simulink model "FlexibleJoint_NNO"  (R2021a)
settings: Solver=VariableStepAuto  StartTime=0.0  StopTime=100  RelTol=1e-3
values from neighbouring files (symbols this model uses):
  A = [[-20 1;0 -20] zeros(2);zeros(2) [-20 1;0 -20]]    [parameters.m]
  Ac = A - G*C    [parameters.m]
  C = eye(4)    [parameters.m]
  eta1 = 1000    [parameters.m]
  eta2 = 1000    [parameters.m]
  G = place(A',C',poles_desired)'    [parameters.m]
  rho1 = 1.5    [parameters.m]
  rho2 = 1.5    [parameters.m]
  size_hiddenlayerneurons = 5    [parameters.m]
  size_systeminput = 1    [parameters.m]
  V0 = 0.1*(2*rand(size_hiddenlayerneurons,size_states + size_systeminput))+100    [parameters.m]
  W0 = 0.1*(2*rand(size_states,size_hiddenlayerneurons))+10    [parameters.m]
settings Model: Creator=kiankhaneghahi  LastModifiedBy=kiankhaneghahi

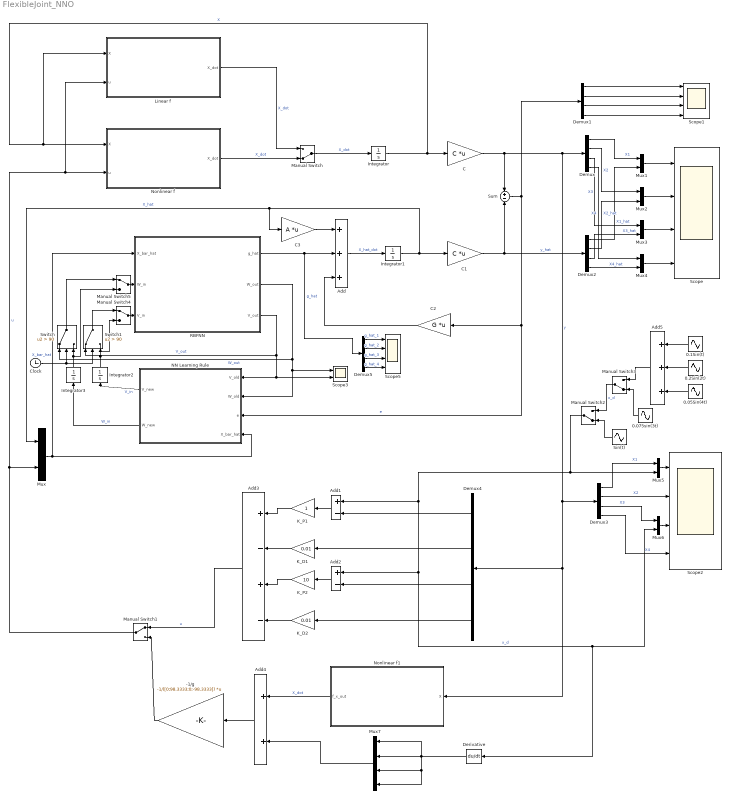
== system FlexibleJoint_NNO ==
  -1/g : Gain  Gain=-1/([0;98.3333;0;-98.3333])  Multiplication=Matrix(K*u)
  0.05Sin(4t) : Sin  Amplitude=0.05  Frequency=4  SampleTime=0
  0.075sin(3t) : Sin  Amplitude=0.075  Frequency=3  SampleTime=0
  0.1Sin(t) : Sin  Amplitude=0.1  SampleTime=0
  0.2Sin(2t) : Sin  Amplitude=0.2  Frequency=2  SampleTime=0
  Add : Sum  Inputs=+++
  Add1 : Sum  Inputs=+-
  Add2 : Sum  Inputs=+-
  Add3 : Sum  Inputs=+-+-
  Add4 : Sum
  Add5 : Sum  Inputs=+++
  C : Gain  Gain=C  Multiplication=Matrix(K*u)
  C1 : Gain  Gain=C  Multiplication=Matrix(K*u)
  C2 : Gain  Gain=G  Multiplication=Matrix(K*u)
  C3 : Gain  Gain=A  Multiplication=Matrix(K*u)
  Clock : Clock
  Demux{,1..5} (6 alike) : Demux
  Derivative : Derivative
  Integrator : Integrator  InitialCondition=[0;0;0;0]
  Integrator1 : Integrator  InitialCondition=[0;0;0;0]
  Integrator2 : Integrator  InitialCondition=V0
  Integrator3 : Integrator  InitialCondition=W0
  K_D1 : Gain  Gain=0.01
  K_D2 : Gain  Gain=0.01
  K_P1 : Gain
  K_P2 : Gain  Gain=10
  Linear f : MATLAB Function  TreatAsAtomicUnit=on
  Manual Switch : ManualSwitch  CurrentSetting=0
  Manual Switch1 : ManualSwitch
  Manual Switch2 : ManualSwitch  CurrentSetting=0
  Manual Switch3 : ManualSwitch  CurrentSetting=0
  Manual Switch4 : ManualSwitch
  Manual Switch5 : ManualSwitch
  Mux{,1..6} (7 alike) : Mux  Inputs=2
  Mux7 : Mux
  NN Learning Rule : MATLAB Function  TreatAsAtomicUnit=on
  Nonlinear f : MATLAB Function  TreatAsAtomicUnit=on
  Nonlinear f1 : MATLAB Function  TreatAsAtomicUnit=on
  RBFNN : MATLAB Function  TreatAsAtomicUnit=on
  Scope{,1..2,5} (4 alike) : Scope  NumInputPorts=4
  Scope3 : Scope  NumInputPorts=2
  Sin(t) : Sin  SampleTime=0
  Sum : Sum  Inputs=+-
  Switch : Switch  Criteria=u2 > Threshold  Threshold=90
  Switch1 : Switch  Criteria=u2 > Threshold  Threshold=90
  wires:
  Integrator/1 -> Linear f/1(X), Nonlinear f/1(X), C/1  "X"
  C3/1 -> Add/1
  NN Learning Rule/1(V_new) -> Integrator2/1  "V_in"
  NN Learning Rule/2(W_new) -> Integrator3/1  "W_in"
  Mux/1 -> NN Learning Rule/4(X_bar_hat), RBFNN/1(X_bar_hat)  "X_bar_hat"
  C1/1 -> Demux2/1, Sum/2  "y_hat"
  Integrator1/1 -> C3/1, Mux/1, C1/1  "X_hat"
  C2/1 -> Add/3
  RBFNN/2(W_out) -> Switch/1, NN Learning Rule/2(W_old), Scope3/1  "W_out"
  Add/1 -> Integrator1/1  "X_hat_dot"
  RBFNN/1(g_hat) -> Demux5/1, Add/2  "g_hat"
  Sum/1 -> Demux1/1, C2/1, NN Learning Rule/3(e)  "e"
  RBFNN/3(V_out) -> NN Learning Rule/1(V_old), Scope3/2, Switch1/1  "V_out"
  C/1 -> Demux4/1, Nonlinear f1/1(X), Demux3/1, Demux/1, Sum/1  "y"
  Manual Switch1/1 -> Linear f/2(u), Nonlinear f/2(u), Mux/2  "u"
  Manual Switch/1 -> Integrator/1  "X_dot"
  Nonlinear f/1(X_dot) -> Manual Switch/2  "X_dot"
  Linear f/1(X_dot) -> Manual Switch/1  "X_dot"
  Demux1/1 -> Scope1/1
  Demux1/2 -> Scope1/2
  Demux1/3 -> Scope1/3
  Demux1/4 -> Scope1/4
  Mux1/1 -> Scope/1
  Mux2/1 -> Scope/2
  Mux3/1 -> Scope/3
  Mux4/1 -> Scope/4
  Demux/1 -> Mux1/1  "X1"
  Demux2/1 -> Mux1/2  "X1_hat"
  Demux/2 -> Mux2/1  "X2"
  Demux2/2 -> Mux2/2  "X2_hat"
  Demux/3 -> Mux3/1  "X3"
  Demux2/3 -> Mux3/2  "X3_hat"
  Demux2/4 -> Mux4/2  "X4_hat"
  Demux/4 -> Mux4/1  "X4"
  Demux3/1 -> Mux5/1  "X1"
  Demux3/2 -> Scope2/2  "X2"
  Demux3/3 -> Mux6/1  "X3"
  Demux3/4 -> Scope2/4  "X4"
  Add1/1 -> K_P1/1
  Demux4/1 -> Add1/2
  Demux4/3 -> Add2/2
  Add2/1 -> K_P2/1
  Demux4/2 -> K_D1/1
  Demux4/4 -> K_D2/1
  K_D1/1 -> Add3/2
  K_D2/1 -> Add3/4
  K_P1/1 -> Add3/1
  K_P2/1 -> Add3/3
  Manual Switch4/1 -> RBFNN/3(V_in)
  Manual Switch5/1 -> RBFNN/2(W_in)
  Mux5/1 -> Scope2/1
  Mux6/1 -> Scope2/3
  Demux5/1 -> Scope5/1  "g_hat_1"
  Demux5/2 -> Scope5/2  "g_hat_2"
  Demux5/3 -> Scope5/3  "g_hat_3"
  Demux5/4 -> Scope5/4  "g_hat_4"
  Add3/1 -> Manual Switch1/1  "u"
  Nonlinear f1/1(f_x_out) -> Add4/1  "X_dot"
  Add4/1 -> -1/g/1
  -1/g/1 -> Manual Switch1/2
  Derivative/1 -> Mux7/3, Mux7/4, Mux7/2, Mux7/1
  Mux7/1 -> Add4/2
  Manual Switch2/1 -> Mux5/2, Derivative/1, Mux6/2, Add2/1, Add1/1  "x_d"
  Sin(t)/1 -> Manual Switch2/2
  Manual Switch3/1 -> Manual Switch2/1  "x_d"
  0.075sin(3t)/1 -> Manual Switch3/2
  Add5/1 -> Manual Switch3/1
  0.1Sin(t)/1 -> Add5/1
  0.2Sin(2t)/1 -> Add5/2
  0.05Sin(4t)/1 -> Add5/3
  Integrator3/1 -> Manual Switch5/2, Switch/3
  Clock/1 -> Switch1/2, Switch/2
  Integrator2/1 -> Manual Switch4/2, Switch1/3
  Switch1/1 -> Manual Switch4/1
  Switch/1 -> Manual Switch5/1

== matlab function FlexibleJoint_NNO/RBFNN ==
  data: X_bar_hat input; g_hat output; W_in input; W_out output; V_in input; V_out output; size_hiddenlayerneurons parameter; size_systeminput parameter
function [g_hat,W_out,V_out] = RBFNN(X_bar_hat, W_in,V_in, size_hiddenlayerneurons, size_systeminput)

m = size_hiddenlayerneurons;               % number of hidden-layer neurons
m_xu = size(X_bar_hat,1);       % input size
m_u = size_systeminput;         % system input size
n = m_xu - m_u;               % output size

% creating the output of the RBF network :

output = zeros(n,1);

for outputindex = 1 : n

    for neuronindex = 1 : m
        
        output(outputindex,1) = output(outputindex,1) + W_in(outputindex,neuronindex) * RBF(X_bar_hat,V_in(neuronindex,:));

    end

end


g_hat = output;
W_out = W_in;
V_out = V_in;
end


function sigma_i = RBF(X_bar_hat,V_i)

    sigma_i = 2/(1 + exp(-2*V_i*X_bar_hat)) -1;

end

== matlab function FlexibleJoint_NNO/Nonlinear f ==
  data: X input; u input; X_dot output
function X_dot = f(X, u)

X1 = X(1,1);
X2 = X(2,1);
X3 = X(3,1);
X4 = X(4,1);

K_s = 1.61;
J_h = 0.0021;
m = 0.403;
g = -9.81;
h = 0.06;
K_m = 0.00767;
K_g = 70;
J_l = 0.0059;
R_m = 2.6;

X1_dot = X2;
X2_dot = - (K_s/J_h)*X1 + (((K_m^2)*(K_g^2))/(R_m*J_h))*X4 - (((K_m)*(K_g))/(R_m*J_h))*u - (K_s/J_l)*X1 + ((m*g*h)/J_l)*sin(X1 + X3);
X3_dot = X4;
X4_dot = (K_s/J_h)*X1 - (((K_m^2)*(K_g^2))/(R_m*J_h))*X4 + (((K_m)*(K_g))/(R_m*J_h))*u;

X_dot = [X1_dot;X2_dot;X3_dot;X4_dot];

end

== matlab function FlexibleJoint_NNO/NN Learning Rule ==
  data: V_old input; V_new output; W_new output; W_old input; e input; X_bar_hat input; Ac parameter; C parameter; size_hiddenlayerneurons parameter; eta1 parameter; eta2 parameter; rho1 parameter; rho2 parameter
function [V_new,W_new] = learningrule(V_old, W_old, e, X_bar_hat, Ac, C, size_hiddenlayerneurons, eta1, eta2, rho1, rho2)


W_hat = W_old;
V_hat = V_old;

Lambda_arg = zeros(1,size_hiddenlayerneurons);
Sigma_hl = zeros(size_hiddenlayerneurons,1);
for m = 1 : size_hiddenlayerneurons
   
    Lambda_arg(1,m) = (RBF(X_bar_hat,V_hat(m,:)))^2;
    Sigma_hl(m,1) = RBF(X_bar_hat,V_hat(m,:));
    
end
Lambda = diag(Lambda_arg);

W_hat_dot = - eta1 * ((e' * C * inv(Ac))') * (Sigma_hl') - rho1*norm(e,2)*W_hat;
V_hat_dot = - eta2 * ((e' * C * inv(Ac) * W_hat * (eye(size_hiddenlayerneurons)-Lambda))') * (sign(X_bar_hat)') - rho2*norm(e,2)*V_hat;

W_hat = W_hat_dot;
V_hat = V_hat_dot;

W_new = W_hat;
V_new = V_hat;

end


function sigma_i = RBF(X_bar_hat,V_i)

    sigma_i = 2/(1 + exp(-2*V_i*X_bar_hat)) -1;

end

== matlab function FlexibleJoint_NNO/Linear f ==
  data: X input; u input; X_dot output
function X_dot = f(X, u)

X1 = X(1,1);
X2 = X(2,1);
X3 = X(3,1);
X4 = X(4,1);

k = 0.8;
J_m = 0.0004;
J_l = 0.0004;
B_m = 0.015;
B_l = 0.001;

X1_dot = X2;
X2_dot = (-1/J_l)*(B_l*X2 + k*(X1 - X3));
X3_dot = X4;
X4_dot = (-1/J_m)*(B_m*X4 - k*(X1 - X3) -u);

X_dot = [X1_dot;X2_dot;X3_dot;X4_dot];
end

== matlab function FlexibleJoint_NNO/Nonlinear f1 ==
  data: X input; f_x_out output
function f_x_out = f_x(X)

X1 = X(1,1);
X2 = X(2,1);
X3 = X(3,1);
X4 = X(4,1);

K_s = 1.61;
J_h = 0.0021;
m = 0.403;
g = -9.81;
h = 0.06;
K_m = 0.00767;
K_g = 70;
J_l = 0.0059;
R_m = 2.6;

X1_dot = X2;
X2_dot = - (K_s/J_h)*X1 + (((K_m^2)*(K_g^2))/(R_m*J_h))*X4 - (K_s/J_l)*X1 + ((m*g*h)/J_l)*sin(X1 + X3);
X3_dot = X4;
X4_dot = (K_s/J_h)*X1 - (((K_m^2)*(K_g^2))/(R_m*J_h))*X4;

f_x_out = [X1_dot;X2_dot;X3_dot;X4_dot];

end
